simulink model "LightCtrl_SWC"  (R2014b)
settings: Solver=FixedStepDiscrete  StartTime=0.0  StopTime=10.0  FixedStep=0.01  RelTol=1e-3
settings Model: Creator=vismrr  LastModifiedBy=vismrr
settings DataIOCC: SaveFormat=StructureWithTime
settings OptimizationCC: ZeroExternalMemoryAtStartup=off  ZeroInternalMemoryAtStartup=off  OptimizeModelRefInitCode=on  LifeSpan=1
settings RTWCC: SystemTargetFile=autosar.tlc  GenCodeOnly=on  TemplateMakefile=ert_default_tmf  Description=AUTOSAR  ProcessScript=autosar_make_rtw_hook
settings CodeAppCC: IgnoreCustomStorageClasses=off
settings STFCustomTargetCC: ParMdlRefBuildCompliant=on  CompOptLevelCompliant=on  IncludeMdlTerminateFcn=off  CombineOutputUpdateFcns=on  SuppressErrorStatus=on  ERTFirstTimeCompliant=on  ERTCustomFileBanners=on  SupportNonFinite=off  SupportComplex=off  SupportContinuousTime=off  SupportNonInlinedSFcns=off  MATLABClassNameForMDSCustomization=Simulink.SoftwareTarget.ERTCustomization  AutosarCompliant=on  GRTInterface=off  SystemTargetFile=autosar.tlc
settings ERTTargetCC: ConcurrentExecutionCompliant=off  IncludeMdlTerminateFcn=off  SuppressErrorStatus=on  SupportNonFinite=off  SupportComplex=off  ModelStepFunctionPrototypeControlCompliant=off  CPPClassGenCompliant=off  AutosarCompliant=on  InlinedParameterPlacement=NonHierarchical  ERTCustomFileTemplate=example_file_process.tlc

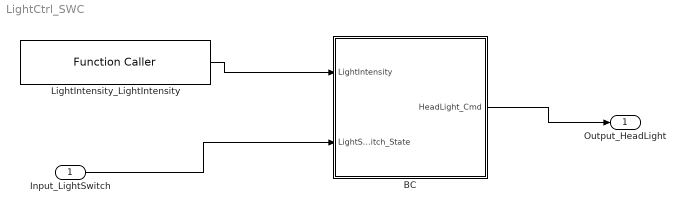
== system LightCtrl_SWC ==
  Input_LightSwitch : Inport  OutDataTypeStr=uint8  PortDimensions=1
  BC : Subsystem  TreatAsAtomicUnit=on
  LightIntensity_LightIntensity : FunctionCaller  FunctionPrototype=io_signal = LightIntensity()  OutputArgumentSpecifications=P_uint16
  Output_HeadLight : Outport  OutDataTypeStr=boolean  PortDimensions=1  SampleTime=0.01
  wires:
  Input_LightSwitch/1 -> BC/2(LightSwitch_State)
  LightIntensity_LightIntensity/1 -> BC/1(LightIntensity)
  BC/1(HeadLight_Cmd) -> Output_HeadLight/1

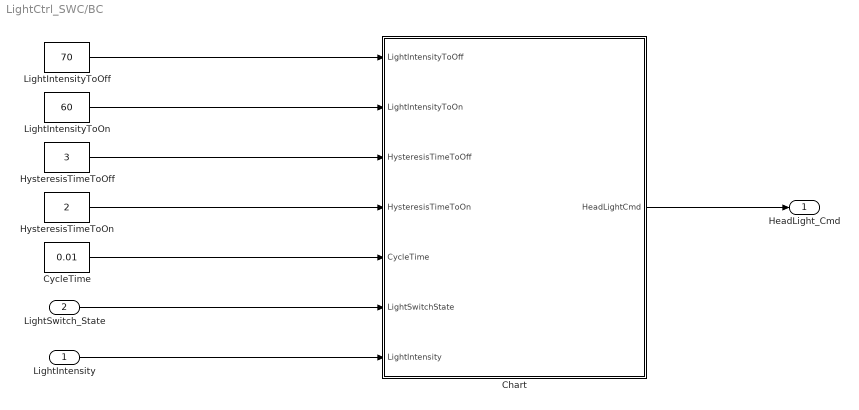
== system LightCtrl_SWC/BC ==
  LightIntensity : Inport
  LightSwitch_State : Inport  Port=2
  Chart : Stateflow chart  TreatAsAtomicUnit=on
  CycleTime : Constant  Value=0.01
  HysteresisTimeToOff : Constant  Value=3
  HysteresisTimeToOn : Constant  Value=2
  LightIntensityToOff : Constant  Value=70
  LightIntensityToOn : Constant  Value=60
  HeadLight_Cmd : Outport
  wires:
  Chart/1(HeadLightCmd) -> HeadLight_Cmd/1
  LightIntensityToOff/1 -> Chart/1(LightIntensityToOff)
  LightIntensityToOn/1 -> Chart/2(LightIntensityToOn)
  HysteresisTimeToOff/1 -> Chart/3(HysteresisTimeToOff)
  HysteresisTimeToOn/1 -> Chart/4(HysteresisTimeToOn)
  CycleTime/1 -> Chart/5(CycleTime)
  LightSwitch_State/1 -> Chart/6(LightSwitchState)
  LightIntensity/1 -> Chart/7(LightIntensity)

== stateflow chart LightCtrl_SWC/BC/Chart ==
  state OffMode
  state AutoMode
    state EnterAutoMode
    state LightOff
    state LightToOn
    state LightToOff
    state LightOn
    (default) -> EnterAutoMode
    EnterAutoMode -> LightOff [order 1] : [LightIntensity>LightIntensityToOff]
    EnterAutoMode -> LightOn [order 2]
    LightOff -> LightOff [order 2] : {HeadLightCmd=0;
        | HysteresisTimer=0;}
    LightToOff -> LightOff [order 2] : [HysteresisTimer>=HysteresisTimeToOff]
    LightOff -> LightToOn [order 1] : [LightIntensity<LightIntensityToOn]
    LightToOn -> LightOff [order 1] : [LightIntensity>=LightIntensityToOn]
    LightToOn -> LightToOn [order 3] : {HysteresisTimer+=CycleTime;}
    LightToOff -> LightOn [order 1] : [LightIntensity<=LightIntensityToOff]
    LightToOff -> LightToOff [order 3] : {HysteresisTimer+=CycleTime;}
    LightToOn -> LightOn [order 2] : [HysteresisTimer>=HysteresisTimeToOn]
    LightOn -> LightToOff [order 1] : [LightIntensity>LightIntensityToOff]
    LightOn -> LightOn [order 2] : {HeadLightCmd=1;
        | HysteresisTimer=0;}
  state OnMode
  (default) -> OffMode
  OffMode -> OffMode [order 3] : {HeadLightCmd=0;}
  OffMode -> AutoMode [order 1] : [LightSwitchState==2]
  OnMode -> OffMode [order 1] : [LightSwitchState==0]
  OffMode -> OnMode [order 2] : [LightSwitchState==1]
  AutoMode -> OffMode [order 2] : [LightSwitchState==0]
  AutoMode -> OnMode [order 1] : [LightSwitchState==1]
  OnMode -> OnMode [order 3] : {HeadLightCmd=1;}
  OnMode -> AutoMode [order 2] : [LightSwitchState==2]
  data: LightIntensityToOff input; LightIntensityToOn input; HysteresisTimeToOff input; HysteresisTimeToOn input; CycleTime input; LightSwitchState input; LightIntensity input; HeadLightCmd output [0..1] =0; HysteresisTimer local double
